simulink model "MIMOprocess_controller"  (Simulink 7.4)
settings: Solver=ode45  StartTime=0.0  StopTime=10.0  RelTol=1e-3
values from neighbouring files (symbols this model uses):
  Kr1 = K_ret(2)    [auslegung.m]
  Kr2 = K_ret(3)    [auslegung.m]
  Kr3 = K_ret(1)    [auslegung.m]
undefined symbols (not defined in the file or in its folder): Kr4, Kr5, Kr6, Kv1, Kv2, Kv3, Kv4
settings Model: Creator=Alex  LastModifiedBy=Alex

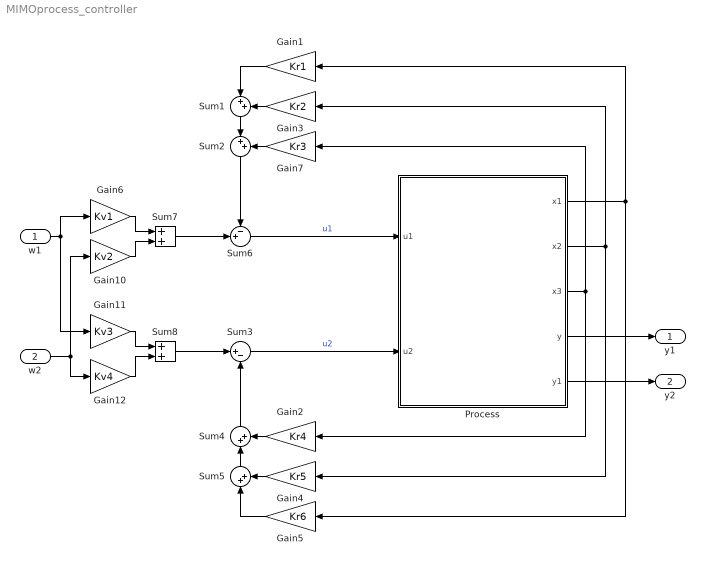
== system MIMOprocess_controller ==
  w1 : Inport  OutDataType=fixdt(1, 16)  OutScaling=2^0
  w2 : Inport  Port=2  OutDataType=fixdt(1, 16)  OutScaling=2^0
  Gain1 : Gain  Gain=Kr1  ParameterDataType=fixdt(1, 16)  ParameterScaling=2^0  OutDataType=fixdt(1, 16)  OutScaling=2^0
  Gain10 : Gain  Gain=Kv2  ParameterDataType=fixdt(1, 16)  ParameterScaling=2^0  OutDataType=fixdt(1, 16)  OutScaling=2^0
  Gain11 : Gain  Gain=Kv3  ParameterDataType=fixdt(1, 16)  ParameterScaling=2^0  OutDataType=fixdt(1, 16)  OutScaling=2^0
  Gain12 : Gain  Gain=Kv4  ParameterDataType=fixdt(1, 16)  ParameterScaling=2^0  OutDataType=fixdt(1, 16)  OutScaling=2^0
  Gain2 : Gain  Gain=Kr4  ParameterDataType=fixdt(1, 16)  ParameterScaling=2^0  OutDataType=fixdt(1, 16)  OutScaling=2^0
  Gain3 : Gain  Gain=Kr2  ParameterDataType=fixdt(1, 16)  ParameterScaling=2^0  OutDataType=fixdt(1, 16)  OutScaling=2^0
  Gain4 : Gain  Gain=Kr5  ParameterDataType=fixdt(1, 16)  ParameterScaling=2^0  OutDataType=fixdt(1, 16)  OutScaling=2^0
  Gain5 : Gain  Gain=Kr6  ParameterDataType=fixdt(1, 16)  ParameterScaling=2^0  OutDataType=fixdt(1, 16)  OutScaling=2^0
  Gain6 : Gain  Gain=Kv1  ParameterDataType=fixdt(1, 16)  ParameterScaling=2^0  OutDataType=fixdt(1, 16)  OutScaling=2^0
  Gain7 : Gain  Gain=Kr3  ParameterDataType=fixdt(1, 16)  ParameterScaling=2^0  OutDataType=fixdt(1, 16)  OutScaling=2^0
  Process : Subsystem
  Sum{1..2,4..5} (4 alike) : Sum  Inputs=|++  OutDataType=fixdt(1, 16)  OutScaling=2^0
  Sum3 : Sum  Inputs=|+-  OutDataType=fixdt(1, 16)  OutScaling=2^0
  Sum6 : Sum  Inputs=-+|  OutDataType=fixdt(1, 16)  OutScaling=2^0
  Sum7 : Sum  OutDataType=fixdt(1, 16)  OutScaling=2^0
  Sum8 : Sum  OutDataType=fixdt(1, 16)  OutScaling=2^0
  y1 : Outport  OutDataType=fixdt(1, 16)  OutScaling=2^0
  y2 : Outport  Port=2  OutDataType=fixdt(1, 16)  OutScaling=2^0
  wires:
  Gain5/1 -> Sum5/1
  Gain4/1 -> Sum5/2
  Gain2/1 -> Sum4/2
  Sum5/1 -> Sum4/1
  Sum4/1 -> Sum3/2
  Process/2(x2) -> Gain4/1, Gain3/1
  w1/1 -> Gain6/1, Gain11/1
  w2/1 -> Gain10/1, Gain12/1
  Gain6/1 -> Sum7/1
  Gain10/1 -> Sum7/2
  Gain11/1 -> Sum8/1
  Gain12/1 -> Sum8/2
  Sum7/1 -> Sum6/2
  Sum8/1 -> Sum3/1
  Process/4(y) -> y1/1
  Process/5(y1) -> y2/1
  Sum6/1 -> Process/1(u1)  "u1"
  Sum3/1 -> Process/2(u2)  "u2"
  Sum1/1 -> Sum2/1
  Sum2/1 -> Sum6/1
  Gain1/1 -> Sum1/1
  Gain3/1 -> Sum1/2
  Gain7/1 -> Sum2/2
  Process/1(x1) -> Gain5/1, Gain1/1
  Process/3(x3) -> Gain2/1, Gain7/1

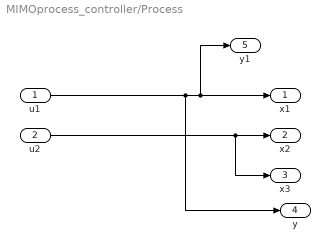
== system MIMOprocess_controller/Process ==
  u1 : Inport  OutDataType=fixdt(1, 16)  OutScaling=2^0
  u2 : Inport  Port=2  OutDataType=fixdt(1, 16)  OutScaling=2^0
  x1 : Outport  OutDataType=fixdt(1, 16)  OutScaling=2^0
  x2 : Outport  Port=2  OutDataType=fixdt(1, 16)  OutScaling=2^0
  x3 : Outport  Port=3  OutDataType=fixdt(1, 16)  OutScaling=2^0
  y : Outport  Port=4  OutDataType=fixdt(1, 16)  OutScaling=2^0
  y1 : Outport  Port=5  OutDataType=fixdt(1, 16)  OutScaling=2^0
  wires:
  u1/1 -> y/1, x1/1, y1/1
  u2/1 -> x2/1, x3/1
